simulink model "orbit_box"  (R2019b)
settings: Solver=ode45  StartTime=0.0  StopTime=20000.0  MaxStep=0.01  RelTol=1e-8
settings Model: Creator=Hector  LastModifiedBy=Hector

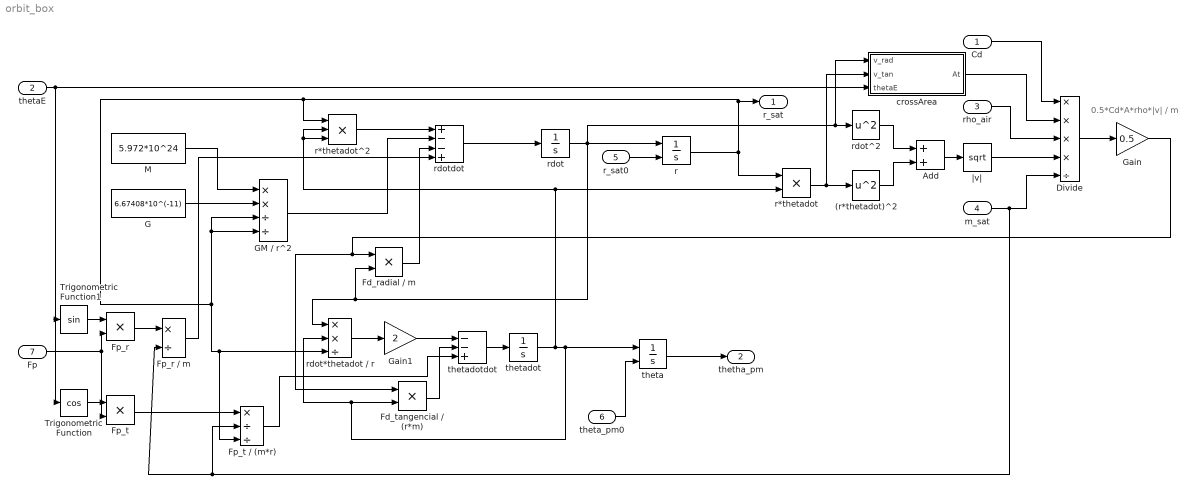
== system orbit_box ==
  note: 0.5*Cd*A*rho*|v| / m
  Cd : Inport
  thetaE : Inport  Port=2
  rho_air : Inport  Port=3
  m_sat : Inport  Port=4
  r_sat0 : Inport  Port=5
  theta_pm0 : Inport  Port=6
  Fp : Inport  Port=7
  (r*thetadot)^2 : Math  Operator=square  SignedPower=off  SaturateOnIntegerOverflow=on
  Add : Sum
  Divide : Product  Inputs=****/
  Fd_radial / m : Product
  "Fd_tangencial / (r*m) " : Product
  Fp_r : Product
  Fp_r / m : Product  Inputs=*/
  Fp_t : Product
  Fp_t / (m*r) : Product  Inputs=*//
  G : Constant  Value=6.67408*10^(-11)
  GM / r^2 : Product  Inputs=**//
  Gain : Gain  Gain=0.5
  Gain1 : Gain  Gain=2
  M : Constant  Value=5.972*10^24
  Trigonometric Function : Trigonometry  Operator=cos
  Trigonometric Function1 : Trigonometry
  crossArea : Subsystem
  r : Integrator  InitialConditionSource=external  InitialCondition=6.7871*10^6
  r*thetadot : Product
  r*thetadot^2 : Product  Inputs=3
  rdot : Integrator
  rdot*thetadot / r : Product  Inputs=**/
  rdot^2 : Math  Operator=square  SignedPower=off  SaturateOnIntegerOverflow=on
  rdotdot : Sum  Inputs=+--+
  theta : Integrator  InitialConditionSource=external  InitialCondition=pi/4
  thetadot : Integrator  InitialCondition=0.001129091743116
  thetadotdot : Sum  Inputs=--+
  |v| : Sqrt  SaturateOnIntegerOverflow=on
  r_sat : Outport
  thetha_pm : Outport  Port=2
  wires:
  Cd/1 -> Divide/1
  rho_air/1 -> Divide/3
  r*thetadot/1 -> crossArea/2(v_tan), (r*thetadot)^2/1
  rdot^2/1 -> Add/1
  (r*thetadot)^2/1 -> Add/2
  Add/1 -> |v|/1
  |v|/1 -> Divide/4
  Divide/1 -> Gain/1
  M/1 -> GM / r^2/1
  G/1 -> GM / r^2/2
  r*thetadot^2/1 -> rdotdot/1
  GM / r^2/1 -> rdotdot/2
  rdotdot/1 -> rdot/1
  Gain/1 -> "Fd_tangencial / (r*m) "/1, Fd_radial / m/1
  Fd_radial / m/1 -> rdotdot/3
  thetadot/1 -> r*thetadot^2/2, r*thetadot^2/3, r*thetadot/2, rdot*thetadot / r/2, "Fd_tangencial / (r*m) "/2, theta/1
  rdot*thetadot / r/1 -> Gain1/1
  Gain1/1 -> thetadotdot/1
  rdot/1 -> crossArea/1(v_rad), rdot^2/1, rdot*thetadot / r/1, Fd_radial / m/2, r/1
  "Fd_tangencial / (r*m) "/1 -> thetadotdot/2
  thetadotdot/1 -> thetadot/1
  r/1 -> r_sat/1, Fp_t / (m*r)/3, rdot*thetadot / r/3, GM / r^2/3, GM / r^2/4, r*thetadot^2/1, r*thetadot/1
  m_sat/1 -> Fp_r / m/2, Fp_t / (m*r)/2, Divide/5
  theta/1 -> thetha_pm/1
  r_sat0/1 -> r/2
  theta_pm0/1 -> theta/2
  thetaE/1 -> crossArea/3(thetaE), Trigonometric Function/1, Trigonometric Function1/1
  crossArea/1(At) -> Divide/2
  Fp_t / (m*r)/1 -> thetadotdot/3
  Fp_r / m/1 -> rdotdot/4
  Trigonometric Function/1 -> Fp_t/1
  Trigonometric Function1/1 -> Fp_r/1
  Fp/1 -> Fp_t/2, Fp_r/2
  Fp_r/1 -> Fp_r / m/1
  Fp_t/1 -> Fp_t / (m*r)/1

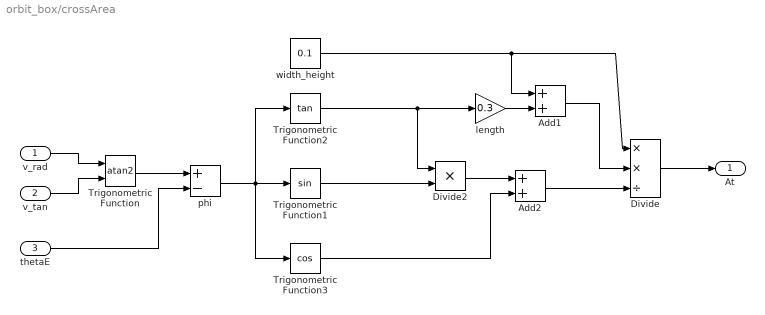
== system orbit_box/crossArea ==
  v_rad : Inport
  v_tan : Inport  Port=2
  thetaE : Inport  Port=3
  Add1 : Sum
  Add2 : Sum
  Divide : Product  Inputs=**/
  Divide2 : Product  Inputs=**
  Trigonometric Function : Trigonometry  Operator=atan2
  Trigonometric Function1 : Trigonometry
  Trigonometric Function2 : Trigonometry  Operator=tan
  Trigonometric Function3 : Trigonometry  Operator=cos
  length : Gain  Gain=0.3
  phi : Sum  Inputs=+-
  width_height : Constant  Value=0.1
  At : Outport
  wires:
  v_rad/1 -> Trigonometric Function/1
  v_tan/1 -> Trigonometric Function/2
  Trigonometric Function/1 -> phi/1
  thetaE/1 -> phi/2
  phi/1 -> Trigonometric Function3/1, Trigonometric Function1/1, Trigonometric Function2/1
  Divide/1 -> At/1
  width_height/1 -> Divide/1, Add1/1
  Trigonometric Function2/1 -> length/1, Divide2/1
  length/1 -> Add1/2
  Add1/1 -> Divide/2
  Trigonometric Function1/1 -> Divide2/2
  Divide2/1 -> Add2/1
  Trigonometric Function3/1 -> Add2/2
  Add2/1 -> Divide/3
